simulink model "test_R2017b"  (R2018b)
settings: Solver=VariableStepAuto  StartTime=0.0  StopTime=600  RelTol=1e-3
values from neighbouring files (symbols this model uses):
  A = jacobian([f1,f2, f3, f4], [x1, x2, x3, x4])    [TaylorRemainder.m]    (also in init_ctrl_design.m = eval(A); init_ctrl_design_simple.m = eval(A))
  Ad = expm(A*dT)    [init_ctrl_design.m]    (also in init_ctrl_design_simple.m = eye(2)+A*Ts)
  AK = Ad-Bd*K    [init_ctrl_design.m]    (also in init_ctrl_design_simple.m)
  B = jacobian([f1,f2, f3, f4], [u])    [TaylorRemainder.m]    (also in init_ctrl_design.m = eval(B); init_ctrl_design_simple.m = eval(B); mgcm_acado.m = 1)
  Bd = (Ad-eye(n))*inv(A)*B    [init_ctrl_design.m]    (also in init_ctrl_design_simple.m = Ts*B)
  beta = 1    [TaylorRemainder.m]    (also in init_ctrl_design.m; init_ctrl_design_simple.m; solveMGCM.m)
  C = eye(4)    [init_ctrl_design.m]    (also in init_ctrl_design_simple.m = eye(2))
  Cd = C    [init_ctrl_design.m]    (also in init_ctrl_design_simple.m = eye(2))
  D = zeros(4,1)    [init_ctrl_design.m]    (also in init_ctrl_design_simple.m = zeros(2,1))
  Dd = D    [init_ctrl_design.m]    (also in init_ctrl_design_simple.m)
  init_cond = [x1-0.35, x2-0.4, x3, 0]    [TaylorRemainder.m]    (also in init_ctrl_design.m; init_ctrl_design_simple.m = [x1-0.35, x2-0.4])
  ksi = 1/sqrt(2)    [solveMGCM.m]
  Ts = 0.01    [APRBSgeneration.m]    (also in draw.m; drawCP.m = 0.1; genTrainingData.m = 0.1; init_ctrl_design.m)
  wn = sqrt(1000)    [TaylorRemainder.m]    (also in init_ctrl_design.m; solveMGCM.m)
  x2_c = 0    [TaylorRemainder.m]    (also in init_ctrl_design.m; init_ctrl_design_simple.m; solveMGCM.m)
settings Model: Creator=pbevanda  LastModifiedBy=pbevanda

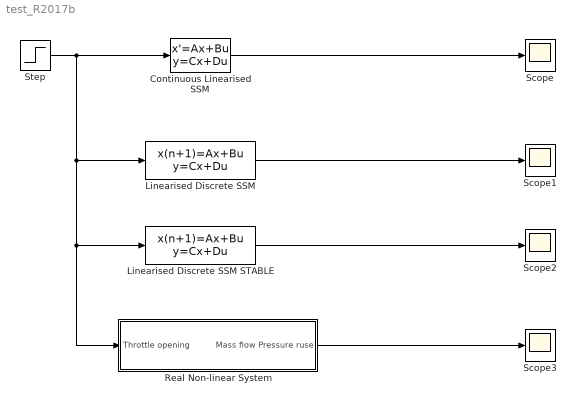
== system test_R2017b ==
  Continuous Linearised SSM : StateSpace  A=A  B=B  C=C  D=D  InitialCondition=init_cond
  "Linearised Discrete SSM " : DiscreteStateSpace  A=Ad  B=Bd  C=Cd  D=Dd  InitialCondition=init_cond  SampleTime=Ts
  Linearised Discrete SSM STABLE : DiscreteStateSpace  A=AK  B=zeros(4,1)  C=Cd  D=Dd  InitialCondition=init_cond  SampleTime=Ts
  "Real Non-linear System " : Subsystem
  Scope{,1..3} (4 alike) : Scope
  Step : Step  Time=0  After=0  SampleTime=0
  wires:
  Continuous Linearised SSM/1 -> Scope/1
  "Linearised Discrete SSM "/1 -> Scope1/1
  Step/1 -> "Real Non-linear System "/1(Throttle opening), Linearised Discrete SSM STABLE/1, "Linearised Discrete SSM "/1, Continuous Linearised SSM/1
  Linearised Discrete SSM STABLE/1 -> Scope2/1
  "Real Non-linear System "/1("Mass flow Pressure ruse ") -> Scope3/1

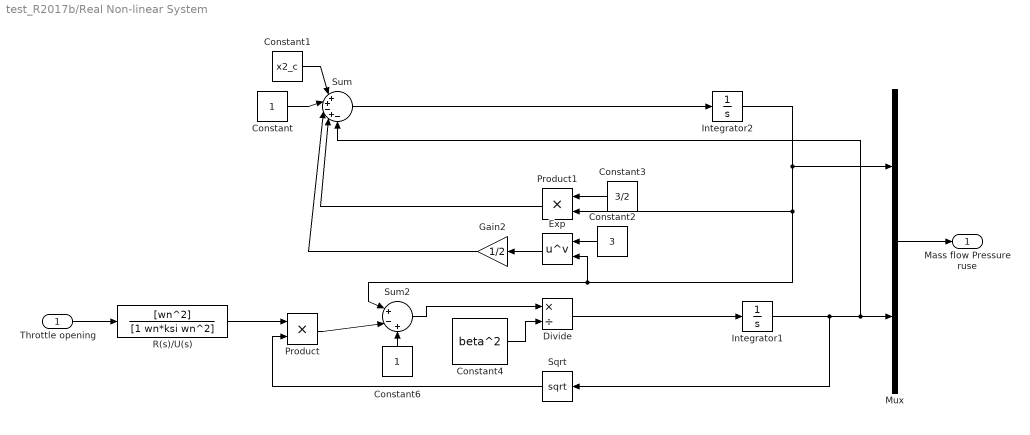
== system test_R2017b/Real Non-linear System  ==
  Throttle opening : Inport
  Constant : Constant
  Constant1 : Constant  Value=x2_c
  Constant2 : Constant  Value=3
  Constant3 : Constant  Value=3/2
  Constant4 : Constant  Value=beta^2
  Constant6 : Constant
  Divide : Product  Inputs=*/
  Exp : Math  Operator=pow  SaturateOnIntegerOverflow=on
  Gain2 : Gain  Gain=1/2
  Integrator1 : Integrator  InitialCondition=init_cond(2)
  Integrator2 : Integrator  InitialCondition=init_cond(1)
  Mux : Mux  Inputs=2
  Product : Product
  Product1 : Product
  R(s)/U(s) : TransferFcn  Numerator=[wn^2]  Denominator=[1 wn*ksi wn^2]
  Sqrt : Sqrt  SaturateOnIntegerOverflow=on
  Sum : Sum  Inputs=|++-+-
  Sum2 : Sum  Inputs=|+-+
  "Mass flow Pressure ruse " : Outport
  wires:
  Mux/1 -> "Mass flow Pressure ruse "/1
  Constant/1 -> Sum/2
  Constant1/1 -> Sum/1
  Throttle opening/1 -> R(s)/U(s)/1
  R(s)/U(s)/1 -> Product/1
  Constant2/1 -> Exp/1
  Constant4/1 -> Divide/2
  Sum2/1 -> Divide/1
  Integrator1/1 -> Sqrt/1, Mux/2, Sum/5
  Integrator2/1 -> Exp/2, Sum2/1, Product1/2, Mux/1
  Constant6/1 -> Sum2/3
  Sqrt/1 -> Product/2
  Product/1 -> Sum2/2
  Divide/1 -> Integrator1/1
  Exp/1 -> Gain2/1
  Gain2/1 -> Sum/3
  Sum/1 -> Integrator2/1
  Constant3/1 -> Product1/1
  Product1/1 -> Sum/4
